simulink model "DTC2018B"  (R2018b)
settings: Solver=VariableStepAuto  StartTime=0.0  StopTime=30  RelTol=1e-3
values from neighbouring files (symbols this model uses):
  Caf = 460    [trqvparameter.m]
  Car = 440    [trqvparameter.m]
  dwf = 1.2    [trqvparameter.m]
  Ki = 5    [trqvparameter.m]
  Kp = 20    [trqvparameter.m]
  lf = 0.761    [trqvparameter.m]
  lr = 0.831    [trqvparameter.m]
  m = 340    [trqvparameter.m]
  Rt = 0.2    [trqvparameter.m]
libraries: simulink x5, Solver_SF x1
settings Model: Creator=12045  LastModifiedBy=12045
settings DataIOCC: ReturnWorkspaceOutputs=on
settings DebuggingCC: UnconnectedInputMsg=none  UnconnectedOutputMsg=none  UnconnectedLineMsg=none  SFMachineParentedDataDiag=error
settings ModelReferenceCC: EnableRefExpFcnMdlSchedulingChecks=off
settings RTWCC: Description=Generic Real-Time Target

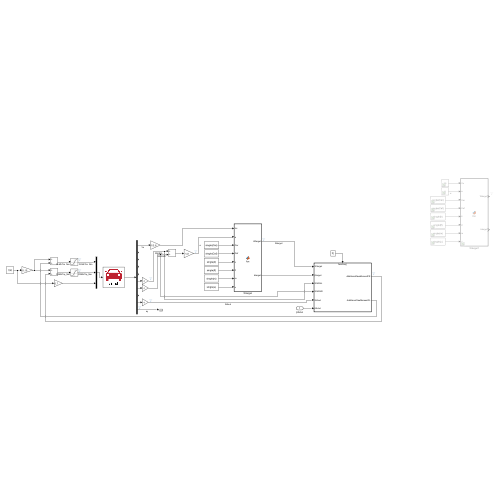
[thumbnail: Simulink's stored preview of the top-level diagram]
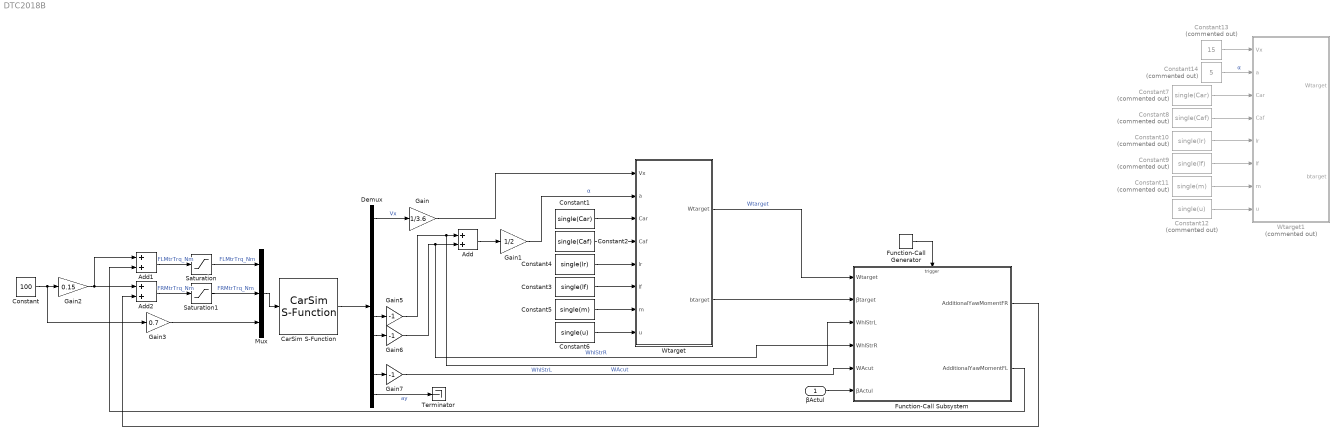
== system DTC2018B ==
  βActul : Inport
  Add : Sum
  Add1 : Sum
  Add2 : Sum
  CarSim S-Function : Solver_SF/CarSim S-Function  Priority=1  SIMFILE=simfile.sim  Run_RTs=off  vs_state_ind=Run  StopMode_ind=Vehicle Model
  Constant : Constant  Value=100
  Constant1 : Constant  Value=single(Car)
  Constant10 : Constant  Commented=on  Value=single(lr)
  Constant11 : Constant  Commented=on  Value=single(m)
  Constant12 : Constant  Commented=on  Value=single(u)
  Constant13 : Constant  Commented=on  Value=15
  Constant14 : Constant  Commented=on  Value=5
  Constant2 : Constant  Value=single(Caf)
  Constant3 : Constant  Value=single(lf)
  Constant4 : Constant  Value=single(lr)
  Constant5 : Constant  Value=single(m)
  Constant6 : Constant  Value=single(u)
  Constant7 : Constant  Commented=on  Value=single(Car)
  Constant8 : Constant  Commented=on  Value=single(Caf)
  Constant9 : Constant  Commented=on  Value=single(lf)
  Demux : Demux  Outputs=10
  Function-Call Generator : simulink/Ports & Subsystems/Function-Call Generator  sample_time=0.01  numberOfIterations=1
  Function-Call Subsystem : Subsystem  TreatAsAtomicUnit=on
  Gain : Gain  Gain=1/3.6
  Gain1 : Gain  Gain=1/2
  Gain2 : Gain  Gain=0.15
  Gain3 : Gain  Gain=0.7
  Gain5 : Gain  Gain=-1
  Gain6 : Gain  Gain=-1
  Gain7 : Gain  Gain=-1
  Mux : Mux  Inputs=3
  Saturation : Saturate  UpperLimit=inf  LowerLimit=0
  Saturation1 : Saturate  UpperLimit=inf  LowerLimit=0
  Terminator : Terminator
  Wtarget : MATLAB Function  TreatAsAtomicUnit=on
  Wtarget1 : MATLAB Function  Commented=on  TreatAsAtomicUnit=on
  wires:
  Gain1/1 -> Wtarget/2(a)  "α"
  Demux/1 -> Gain/1  "Vx"
  Function-Call Generator/1 -> Function-Call Subsystem/Trigger
  Wtarget/1(Wtarget) -> Function-Call Subsystem/1(Wtarget)  "Wtarget"
  Wtarget/2(btarget) -> Function-Call Subsystem/2(βtarget)
  Demux/9 -> Gain7/1
  βActul/1 -> Function-Call Subsystem/6(βActul)
  Function-Call Subsystem/1(AdditionalYawMomentFR) -> Add2/2
  CarSim S-Function/1 -> Demux/1
  Demux/6 -> Gain5/1
  Demux/7 -> Gain6/1
  Add/1 -> Gain1/1
  Gain7/1 -> Function-Call Subsystem/5(WAcut)  "WAcut"
  Mux/1 -> CarSim S-Function/1
  Constant/1 -> Gain3/1, Gain2/1
  Gain3/1 -> Mux/3
  Add1/1 -> Saturation/1  "FLMtrTrq_Nm"
  Add2/1 -> Saturation1/1  "FRMtrTrq_Nm"
  Gain2/1 -> Add1/1, Add2/1
  Saturation/1 -> Mux/1  "FLMtrTrq_Nm"
  Saturation1/1 -> Mux/2  "FRMtrTrq_Nm"
  Gain5/1 -> Function-Call Subsystem/3(WhlStrL), Add/1  "WhlStrL"
  Gain6/1 -> Add/2, Function-Call Subsystem/4(WhlStrR)  "WhlStrR"
  Gain/1 -> Wtarget/1(Vx)
  Constant5/1 -> Wtarget/7(m)
  Constant6/1 -> Wtarget/8(u)
  Constant4/1 -> Wtarget/5(lr)
  Constant2/1 -> Wtarget/4(Caf)
  Constant1/1 -> Wtarget/3(Car)
  Constant3/1 -> Wtarget/6(lf)
  Constant9/1 -> Wtarget1/6(lf)
  Constant7/1 -> Wtarget1/3(Car)
  Constant8/1 -> Wtarget1/4(Caf)
  Constant10/1 -> Wtarget1/5(lr)
  Constant12/1 -> Wtarget1/8(u)
  Constant11/1 -> Wtarget1/7(m)
  Constant13/1 -> Wtarget1/1(Vx)
  Constant14/1 -> Wtarget1/2(a)  "α"
  Function-Call Subsystem/2(AdditionalYawMomentFL) -> Add1/2
  Demux/10 -> Terminator/1  "ay"

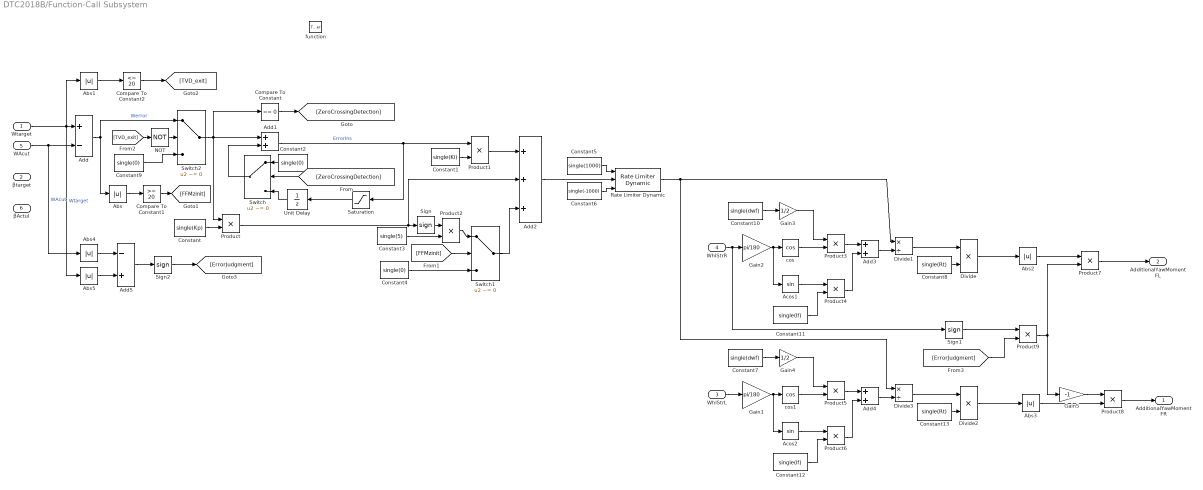
== system DTC2018B/Function-Call Subsystem ==
  Wtarget : Inport
  βtarget : Inport  Port=2
  WhlStrL : Inport  Port=3
  WhlStrR : Inport  Port=4
  WAcut : Inport  Port=5
  βActul : Inport  Port=6
  function : TriggerPort  TriggerType=function-call  VariantControl=(inherit)
  Abs{,1..5} (6 alike) : Abs
  Acos1 : Trigonometry
  Acos2 : Trigonometry
  Add : Sum  Inputs=+-
  Add1 : Sum
  Add2 : Sum  Inputs=+++
  Add3 : Sum
  Add4 : Sum
  Add5 : Sum  Inputs=-+
  Compare To Constant : simulink/Logic and Bit Operations/Compare To Constant  relop===  const=0  OutDataTypeStr=boolean
  Compare To Constant1 : simulink/Logic and Bit Operations/Compare To Constant  relop=>=  const=20  OutDataTypeStr=boolean
  Compare To Constant2 : simulink/Logic and Bit Operations/Compare To Constant  relop=<=  const=20  OutDataTypeStr=boolean
  Constant : Constant  Value=single(Kp)
  Constant1 : Constant  Value=single(Ki)
  Constant10 : Constant  Value=single(dwf)
  Constant11 : Constant  Value=single(lf)
  Constant12 : Constant  Value=single(lf)
  Constant13 : Constant  Value=single(Rt)
  Constant2 : Constant  Value=single(0)
  Constant3 : Constant  Value=single(5)
  Constant4 : Constant  Value=single(0)
  Constant5 : Constant  Value=single(1000)
  Constant6 : Constant  Value=single(-1000)
  Constant7 : Constant  Value=single(dwf)
  Constant8 : Constant  Value=single(Rt)
  Constant9 : Constant  Value=single(0)
  Divide : Product  Inputs=**
  Divide1 : Product  Inputs=*/
  Divide2 : Product  Inputs=**
  Divide3 : Product  Inputs=*/
  Gain1 : Gain  Gain=pi/180
  Gain2 : Gain  Gain=pi/180
  Gain3 : Gain  Gain=1/2
  Gain4 : Gain  Gain=1/2
  Gain5 : Gain  Gain=-1
  NOT : Logic  Operator=NOT  AllPortsSameDT=off  OutDataTypeStr=boolean
  Product{,1..9} (10 alike) : Product
  Rate Limiter Dynamic : simulink/Discontinuities/Rate Limiter Dynamic
  Saturation : Saturate  UpperLimit=10  LowerLimit=-10
  Sign : Signum
  Sign1 : Signum
  Sign2 : Signum
  Switch : Switch  Criteria=u2 ~= 0
  Switch1 : Switch  Criteria=u2 ~= 0
  Switch2 : Switch  Criteria=u2 ~= 0
  Unit Delay : UnitDelay  SampleTime=-1  HasFrameUpgradeWarning=on
  cos : Trigonometry  Operator=cos
  cos1 : Trigonometry  Operator=cos
  AdditionalYawMomentFR : Outport
  AdditionalYawMomentFL : Outport  Port=2
  wires:
  Wtarget/1 -> Abs5/1, Abs1/1, Add/1  "Wtarget"
  WAcut/1 -> Abs4/1, Add/2  "WAcut"
  Add/1 -> Abs/1, Switch2/1  "Werror"
  Constant/1 -> Product/2
  Add1/1 -> Saturation/1, Product1/1  "ErrorIns"
  Constant1/1 -> Product1/2
  Product1/1 -> Add2/1
  Product/1 -> Add2/2, Sign/1
  Saturation/1 -> Unit Delay/1
  Switch/1 -> Add1/2
  Constant2/1 -> Switch/1
  Unit Delay/1 -> Switch/3
  Compare To Constant/1 -> [ZeroCrossingDetection]
  [ZeroCrossingDetection] -> Switch/2
  Switch1/1 -> Add2/3
  Compare To Constant1/1 -> [FFMzinit]
  [FFMzinit] -> Switch1/2
  Constant4/1 -> Switch1/3
  Constant8/1 -> Divide/2
  Abs/1 -> Compare To Constant1/1
  Constant3/1 -> Product2/2
  Product2/1 -> Switch1/1
  Sign/1 -> Product2/1
  Constant5/1 -> Rate Limiter Dynamic/1
  Constant6/1 -> Rate Limiter Dynamic/3
  Abs1/1 -> Compare To Constant2/1
  Compare To Constant2/1 -> [TVD_exit]
  Switch2/1 -> Compare To Constant/1, Product/1, Add1/1
  [TVD_exit] -> NOT/1
  NOT/1 -> Switch2/2
  Constant9/1 -> Switch2/3
  WhlStrR/1 -> Sign1/1, Gain2/1
  Gain2/1 -> Acos1/1, cos/1
  Constant10/1 -> Gain3/1
  cos/1 -> Product3/2
  Gain3/1 -> Product3/1
  Product3/1 -> Add3/1
  Acos1/1 -> Product4/1
  Constant11/1 -> Product4/2
  Product4/1 -> Add3/2
  Add3/1 -> Divide1/2
  Divide1/1 -> Divide/1
  Divide/1 -> Abs2/1
  Divide3/1 -> Divide2/1
  Add4/1 -> Divide3/2
  Product6/1 -> Add4/2
  Constant12/1 -> Product6/2
  Acos2/1 -> Product6/1
  Product5/1 -> Add4/1
  Gain4/1 -> Product5/1
  cos1/1 -> Product5/2
  Constant7/1 -> Gain4/1
  Gain1/1 -> cos1/1, Acos2/1
  WhlStrL/1 -> Gain1/1
  Rate Limiter Dynamic/1 -> Divide3/1, Divide1/1
  Constant13/1 -> Divide2/2
  Divide2/1 -> Abs3/1
  Product7/1 -> AdditionalYawMomentFL/1
  Product8/1 -> AdditionalYawMomentFR/1
  Add2/1 -> Rate Limiter Dynamic/2
  Abs2/1 -> Product7/1
  Abs3/1 -> Product8/2
  Sign2/1 -> [ErrorJudgment]
  [ErrorJudgment] -> Product9/2
  Sign1/1 -> Product9/1
  Product9/1 -> Product7/2, Gain5/1
  Gain5/1 -> Product8/1
  Abs4/1 -> Add5/1
  Abs5/1 -> Add5/2
  Add5/1 -> Sign2/1

== matlab function DTC2018B/Wtarget1 ==
  data: Vx input size=1; Wtarget output size=1; a input size=1; Car input size=1; Caf input size=1; lr input size=1; lf input size=1; m input; u input; btarget output
function [Wtarget,btarget] = fcn(Vx,a,Car,Caf,lr,lf,m,u)
Wdes = Vx*a/(lf+lr+(m*Vx*Vx*(lr*Car-lf*Caf)/(Caf*Car*(lr+lf)*2)));
Wu = 0.85*u*9.8/Vx;
if abs(Wdes)<=Wu
Wtarget = Wdes;
else
    Wtarget = Wu*sign(Wdes);
end
bdes = (lr-lf*m*Vx*Vx/Car/(lf+lr)/2)*a/(lr+lf+m*Vx*Vx*(lr*Car-lf*Caf)/Car/Caf/(lf+lr)/2);
bu = atan(0.02*u*9.8);
if abs(bdes)<=bu
btarget = bdes;
else
    btarget = bu*sign(bdes);
end

== matlab function DTC2018B/Wtarget ==
  data: Vx input size=1; Wtarget output size=1; a input size=1; Car input size=1; Caf input size=1; lr input size=1; lf input size=1; m input; u input; btarget output
function [Wtarget,btarget] = fcn(Vx,a,Car,Caf,lr,lf,m,u)
Wdes = Vx*a/(lf+lr+(m*Vx*Vx*(lr*Car-lf*Caf)/Caf/Car/(lr+lf)/2));
Wu = 0.85*u*9.8/Vx;
%if abs(Wdes)<=Wu
Wtarget = Wdes;
%else
 %   Wtarget = Wu*sign(Wdes);
%end
bdes = (lr-lf*m*Vx*Vx/Car/(lf+lr)/2)*a/(lr+lf+m*Vx*Vx*(lr*Car-lf*Caf)/Car/Caf/(lf+lr)/2);
bu = atan(0.02*u*9.8);
if abs(bdes)<=bu
btarget = bdes;
else
    btarget = bu*sign(bdes);
end
